simulink model "advanced_robotics_control"  (R2024a)
settings: Solver=ode1  StartTime=0.0  StopTime=10  FixedStep=0.01  RelTol=1e-3
settings Model: Creator=gujun  LastModifiedBy=gujun
settings RTWCC: GPUComputeCapability=3.5

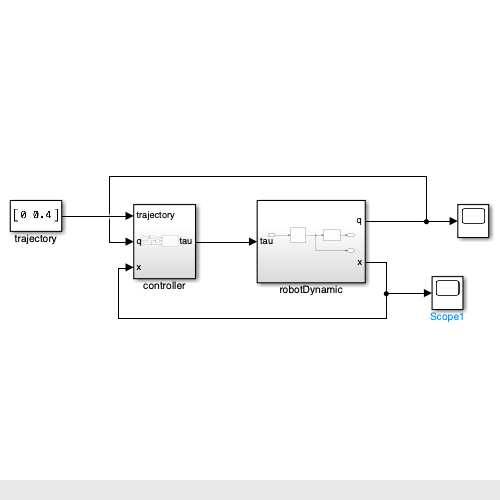
[thumbnail: Simulink's stored preview of the top-level diagram]
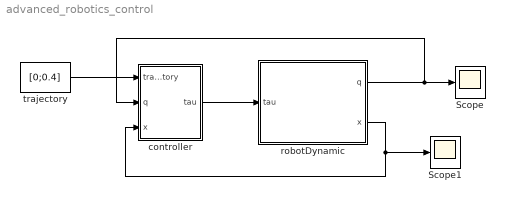
== system advanced_robotics_control ==
  Scope : Scope
  Scope1 : Scope
  controller : Subsystem
  robotDynamic : Subsystem
  trajectory : Constant  Value=[0;0.4]
  wires:
  robotDynamic/1(q) -> controller/2(q), Scope/1
  trajectory/1 -> controller/1(trajectory)
  controller/1(tau) -> robotDynamic/1(tau)
  robotDynamic/2(x) -> Scope1/1, controller/3(x)

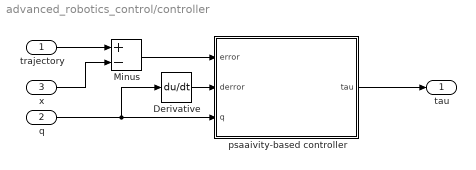
== system advanced_robotics_control/controller ==
  trajectory : Inport
  q : Inport  Port=2
  x : Inport  Port=3
  Derivative : Derivative
  Minus : Sum  Inputs=+-
  psaaivity-based controller : MATLAB Function  TreatAsAtomicUnit=on
  tau : Outport
  wires:
  trajectory/1 -> Minus/1
  x/1 -> Minus/2
  q/1 -> psaaivity-based controller/3(q), Derivative/1
  Derivative/1 -> psaaivity-based controller/2(derror)
  psaaivity-based controller/1(tau) -> tau/1
  Minus/1 -> psaaivity-based controller/1(error)

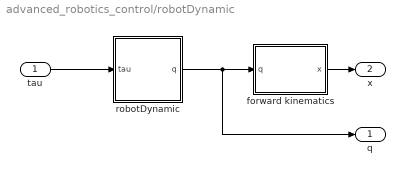
== system advanced_robotics_control/robotDynamic ==
  tau : Inport
  forward kinematics : MATLAB Function  TreatAsAtomicUnit=on
  robotDynamic : Subsystem
  q : Outport
  x : Outport  Port=2
  wires:
  forward kinematics/1(x) -> x/1
  tau/1 -> robotDynamic/1(tau)
  robotDynamic/1(q) -> q/1, forward kinematics/1(q)

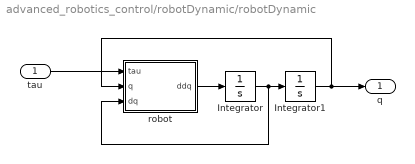
== system advanced_robotics_control/robotDynamic/robotDynamic ==
  tau : Inport
  Integrator : Integrator
  Integrator1 : Integrator
  robot : MATLAB Function  TreatAsAtomicUnit=on
  q : Outport
  wires:
  robot/1(ddq) -> Integrator/1
  tau/1 -> robot/1(tau)
  Integrator1/1 -> q/1, robot/2(q)
  Integrator/1 -> Integrator1/1, robot/3(dq)

== matlab function advanced_robotics_control/robotDynamic/robotDynamic/robot ==
  data: tau input size=2; ddq output size=2; q input size=2; dq input size=2
function ddq = robot(tau, q, dq)

I1 = 0.05;
m1 = 1.5;
lg1 = 0.2;
lr1 = lg1 / 2;

I2 = 0.01;
m2 = 0.5;
lg2 = 0.2;
lr2 = lg2 / 2;

g = 9.8;

M = [m1 * lr1^2 + I1 + m2 * lg1^2, m2 * lg1 * lr2 * cos(q(2));
        m2 * lg1 * lr2 * cos(q(2)), m2 * lr2^2 + I2];

V = [-m2 * lg1 * lr2 * dq(2)^2 * sin(q(2));
    m2 * lg1 * lr2 * dq(1)^2 * sin(q(2))];

G = [m1 * g * lr1 * cos(q(1)) + m2 * g * lg1 * cos(q(1));
    m2 * g * lr2 * cos(q(1) + q(2));];

ddq = M \ (tau - V - G);

end

== matlab function advanced_robotics_control/controller/psaaivity-based controller ==
  data: error input size=2; tau output size=2; derror input size=2; q input size=2
function tau = controller(error, derror, q)

lg1 = 0.2;
lg2 = 0.2;

kp = [0, 0;
       0, 0];


kd = [0, 0;
        0, 0];

jacobian = [-lg1 * sin(q(1)) - lg2 * sin(q(1) + q(2)), -lg2 * sin(q(1) + q(2));
    lg1 * cos(q(1)) + lg2 * cos(q(1) + q(2)), lg2 * cos(q(1) + q(2))];


tau = kp * transpose(jacobian) * error - kd * derror;
end

== matlab function advanced_robotics_control/robotDynamic/forward kinematics ==
  data: q input; x output
function x = kinematics(q)

lg1 = 0.2;
lg2 = 0.2;
x = [0;
    0];
x(1) = lg1 * cos(q(1)) + lg2 * cos(q(1) + q(2));
x(2) = lg1 * sin(q(1)) + lg2 * sin(q(1) + q(2));

end
